simulink subsystem "multirotor_dynamic_model_sim"  (R2023b)
settings: Solver=VariableStepAuto  StartTime=0.0  StopTime=10.0  RelTol=1e-3
settings Model: Creator=minu_  LastModifiedBy=minu_

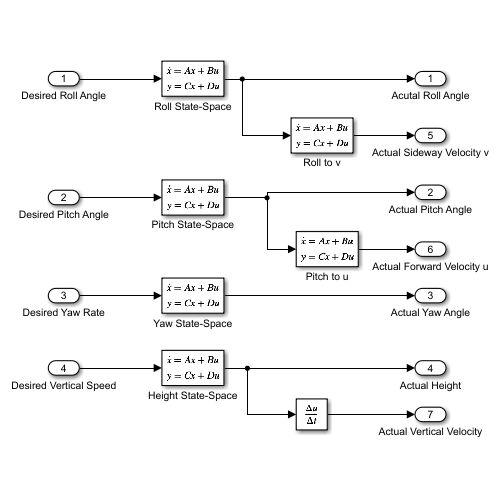
[thumbnail: Simulink's stored preview of the top-level diagram]
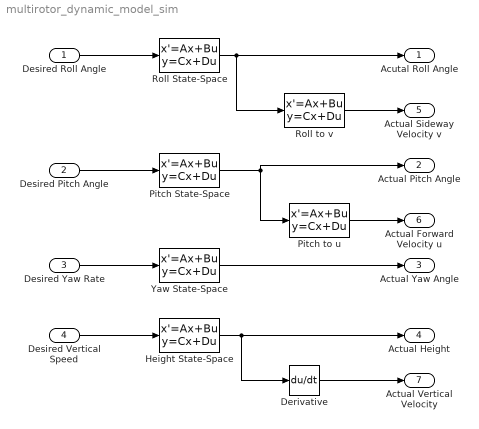
== system multirotor_dynamic_model_sim ==
  Desired Roll Angle : Inport
  Desired Pitch Angle : Inport  Port=2
  Desired Yaw Rate : Inport  Port=3
  Desired Vertical Speed : Inport  Port=4
  Derivative : Derivative
  Height State-Space : StateSpace  A=[-5.8200 -3.6046e-6; 3.8147e-6 0]  B=[1024; 0]  C=[1.4907e-4 1.3191e3]  D=0  InitialCondition=0
  Pitch State-Space : StateSpace  A=[-3.9784 -2.9796; 4 0]  B=[2; 0]  C=[1.2569 0.6083]  D=0  InitialCondition=0
  Pitch to u : StateSpace  A=[-0.665]  B=[2]  C=[-3.0772]  D=0  InitialCondition=0
  Roll State-Space : StateSpace  A=[-4.2683 -3.1716; 4 0]  B=[2; 0]  C=[0.7417 0.4405]  D=0  InitialCondition=0
  Roll to v : StateSpace  A=[-0.4596]  B=[2]  C=[2.3868]  D=0  InitialCondition=0
  Yaw State-Space : StateSpace  A=[-0.0059]  B=[1]  C=[1.2653]  D=0  InitialCondition=0
  Acutal Roll Angle : Outport
  Actual Pitch Angle : Outport  Port=2
  Actual Yaw Angle : Outport  Port=3
  Actual Height : Outport  Port=4
  Actual Sideway Velocity v : Outport  Port=5
  Actual Forward Velocity u : Outport  Port=6
  Actual Vertical Velocity : Outport  Port=7
  wires:
  Pitch State-Space/1 -> Pitch to u/1, Actual Pitch Angle/1
  Derivative/1 -> Actual Vertical Velocity/1
  Roll State-Space/1 -> Roll to v/1, Acutal Roll Angle/1
  Desired Pitch Angle/1 -> Pitch State-Space/1
  Desired Vertical Speed/1 -> Height State-Space/1
  Desired Yaw Rate/1 -> Yaw State-Space/1
  Desired Roll Angle/1 -> Roll State-Space/1
  Height State-Space/1 -> Derivative/1, Actual Height/1
  Pitch to u/1 -> Actual Forward Velocity u/1
  Roll to v/1 -> Actual Sideway Velocity v/1
  Yaw State-Space/1 -> Actual Yaw Angle/1
